simulink model "Microgrid_System"  (R2023b)
settings: Solver=ode23t  StartTime=0.0  StopTime=15.0  RelTol=1e-3
libraries: spsGroundLib x5, spsControlledCurrentSourceLib x4, eeGeneralControl x3, spsPowerLib x3, spsACVoltageSourceLib x1, spsCurrentMeasurementLib x1, spsParallelRLCLoadLib x1, spsSeriesRLCBranchLib x1, spsVoltageMeasurementLib x1, spspowerguiLib x1
settings Model: Creator=Ekta kumari khanda  LastModifiedBy=Ekta kumari khanda

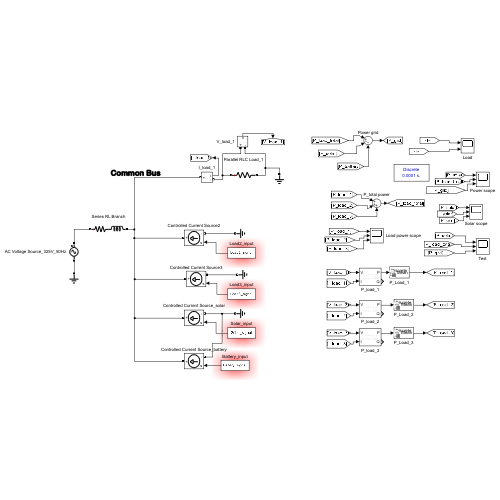
[thumbnail: Simulink's stored preview of the top-level diagram]
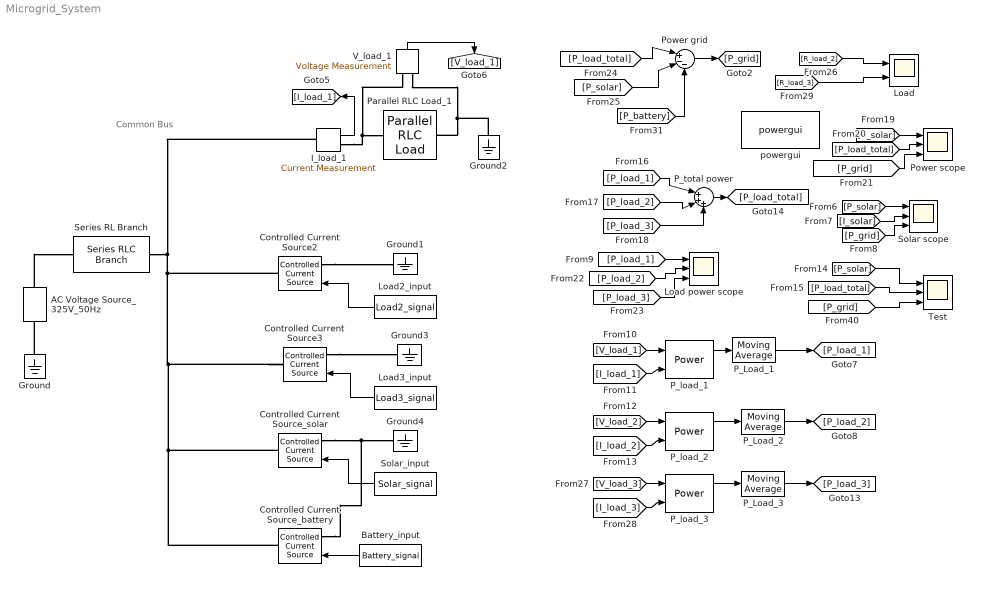
== system Microgrid_System ==
  note: Common Bus
  AC Voltage Source_325V_50Hz : spsACVoltageSourceLib/AC Voltage Source  Amplitude=325  Phase=0  Frequency=50  SampleTime=0  Measurements=None  BusType=swing  Pref=10e3  Qref=0  Qmin=-inf  Qmax=+inf
  Battery_input : FromWorkspace  VariableName=Battery_signal  SampleTime=-1  OutputAfterFinalValue=Holding final value
  Controlled Current Source2 : spsControlledCurrentSourceLib/Controlled Current Source  Initialize=on  Source_Type=AC  Amplitude=0  Phase=0  Frequency=0  Measurements=None
  Controlled Current Source3 : spsControlledCurrentSourceLib/Controlled Current Source  Initialize=on  Source_Type=AC  Amplitude=0  Phase=0  Frequency=0  Measurements=None
  Controlled Current Source_battery : spsControlledCurrentSourceLib/Controlled Current Source  Initialize=on  Source_Type=AC  Amplitude=0  Phase=0  Frequency=0  Measurements=None
  Controlled Current Source_solar : spsControlledCurrentSourceLib/Controlled Current Source  Initialize=on  Source_Type=AC  Amplitude=0  Phase=0  Frequency=0  Measurements=None
  Ground{,1..4} (5 alike) : spsGroundLib/Ground  LConnTagsString=a
  I_load_1 : spsCurrentMeasurementLib/Current Measurement  PhasorSimulation=off  OutputType=Complex  PSBequivalent=0
  Load : Scope  NumInputPorts=2
  Load power scope : Scope  NumInputPorts=3
  Load2_input : FromWorkspace  VariableName=Load2_signal  SampleTime=-1  OutputAfterFinalValue=Holding final value
  Load3_input : FromWorkspace  VariableName=Load3_signal  SampleTime=-1  OutputAfterFinalValue=Holding final value
  P_Load_1 : eeGeneralControl/Moving Average  VariantControl=Variant1  LabelModeActiveChoice=Discrete  f=50  x0=0  BufferSize=8192  Ts=0.001
      settings: LibrarySourceBlock=ee_sl_lib/General Control/Moving Average
  P_Load_2 : eeGeneralControl/Moving Average  VariantControl=Variant1  LabelModeActiveChoice=Discrete  f=50  x0=0  BufferSize=8192  Ts=0.001
      settings: LibrarySourceBlock=ee_sl_lib/General Control/Moving Average
  P_Load_3 : eeGeneralControl/Moving Average  VariantControl=Variant1  LabelModeActiveChoice=Discrete  f=50  x0=0  BufferSize=8192  Ts=0.001
      settings: LibrarySourceBlock=ee_sl_lib/General Control/Moving Average
  P_load_1 : spsPowerLib/Power  Freq=60  Vinit=[1, 0]  Iinit=[1, 0]  Ts=0
  P_load_2 : spsPowerLib/Power  Freq=60  Vinit=[1, 0]  Iinit=[1, 0]  Ts=0
  P_load_3 : spsPowerLib/Power  Freq=60  Vinit=[1, 0]  Iinit=[1, 0]  Ts=0
  P_total power : Sum  Inputs=|+++
  Parallel RLC Load_1 : spsParallelRLCLoadLib/Parallel RLC Load  LConnTagsString=a  RConnTagsString=__new0  NominalVoltage=230  NominalFrequency=50  ActivePower=1500  InductivePower=0  CapacitivePower=0  Setx0=off  InitialVoltage=0  SetiL0=off  InitialCurrent=0  Measurements=None  LoadType=constant Z
      settings: AttributesFormatString=\n  LibrarySourceBlock=sps_lib/Passives/Parallel RLC Load
  Power grid : Sum  Inputs=|+--
  Power scope : Scope  NumInputPorts=3
  Series RL Branch : spsSeriesRLCBranchLib/Series RLC Branch  LConnTagsString=__new0  RConnTagsString=__new0  BranchType=RL  Resistance=0.5  Inductance=1e-3  SetiL0=off  InitialCurrent=0  Capacitance=1e-6  Setx0=off  InitialVoltage=0  Measurements=None
  Solar scope : Scope  NumInputPorts=3
  Solar_input : FromWorkspace  VariableName=Solar_signal  SampleTime=-1  OutputAfterFinalValue=Holding final value
  Test : Scope  NumInputPorts=3
  V_load_1 : spsVoltageMeasurementLib/Voltage Measurement  PhasorSimulation=off  OutputType=Complex  PSBequivalent=0
  powergui : spspowerguiLib/powergui  Priority=1  SimulationMode=Discrete  SampleTime=0.0001  frequency=60  Iterations=50  frequencyindice=0  Pbase=100e6  ErrMax=1e-4  UnitsV=kV  UnitsW=MW  buscounter=0  FunctionMessages=off  echomessages=off  EnableUseOfTLC=off  CurrentSourceSwitches=off  DisableSnubberDevices=off  DisableRonSwitches=off  DisableVfSwitches=off  DisplayEquations=off  AutomaticDiscreteSolvers=off  SolverType=Tustin/Backward Euler (TBE)  Interpol=off  ExternalGateDelay=off  methode=off  Ts=100  x0status=blocks  SPID=on  SwTol=0  HookPort=off  NonlinearTolerance=1e-4  nMaxIteration=100  ContinueOnMaxIteration=off  RestoreLinks=warning  ResistiveCurrentMeasurement=off  Frange=[0:2:500]  Ylog=off  Xlog=on  ShowGrid=off  save=off  variable=ZData  structure=0  ZoomFFT=off  StartTime=0.0  cycles=1  DisplayStyle=1  fundamental=60  FreqAxis=off  MaxFrequency=1000  frequencyindicesteady=1  RmsSteady=1  display=off
  wires:
  [P_solar] -> Solar scope/1
  [P_grid] -> Solar scope/3
  [I_solar] -> Solar scope/2
  I_load_1/1 -> [I_load_1]
  V_load_1/1 -> [V_load_1]
  [I_load_1] -> P_load_1/2
  [V_load_1] -> P_load_1/1
  [V_load_2] -> P_load_2/1
  P_load_2/1 -> P_Load_2/1
  [I_load_2] -> P_load_2/2
  P_Load_2/1 -> [P_load_2]
  [P_load_1] -> P_total power/1
  [P_load_2] -> P_total power/2
  [P_load_3] -> P_total power/3
  P_total power/1 -> [P_load_total]
  [P_solar] -> Power scope/1
  [P_grid] -> Power scope/3
  [P_load_total] -> Power scope/2
  [P_load_3] -> Load power scope/3
  [P_load_2] -> Load power scope/2
  [P_load_1] -> Load power scope/1
  P_Load_1/1 -> [P_load_1]
  P_load_1/1 -> P_Load_1/1
  [P_load_total] -> Test/2
  [P_solar] -> Test/1
  [P_grid] -> Test/3
  P_Load_3/1 -> [P_load_3]
  [I_load_3] -> P_load_3/2
  P_load_3/1 -> P_Load_3/1
  [V_load_3] -> P_load_3/1
  [R_load_2] -> Load/1
  [R_load_3] -> Load/2
  Load2_input/1 -> Controlled Current Source2/1
  Load3_input/1 -> Controlled Current Source3/1
  Solar_input/1 -> Controlled Current Source_solar/1
  Power grid/1 -> [P_grid]
  [P_load_total] -> Power grid/1
  [P_solar] -> Power grid/2
  Battery_input/1 -> Controlled Current Source_battery/1
  [P_battery] -> Power grid/3
  connections:
  Ground/LConn1 -- AC Voltage Source_325V_50Hz/LConn1
  I_load_1/RConn1 -- Parallel RLC Load_1/LConn1 -- V_load_1/LConn1
  V_load_1/LConn2 -- Ground2/LConn1 -- Parallel RLC Load_1/RConn1
  AC Voltage Source_325V_50Hz/RConn1 -- Series RL Branch/LConn1
  Series RL Branch/RConn1 -- I_load_1/LConn1 -- Controlled Current Source_solar/RConn1 -- Controlled Current Source_battery/RConn1 -- Controlled Current Source3/RConn1 -- Controlled Current Source2/RConn1
  Controlled Current Source3/LConn1 -- Ground3/LConn1
  Controlled Current Source2/LConn1 -- Ground1/LConn1
  Controlled Current Source_solar/LConn1 -- Controlled Current Source_battery/LConn1 -- Ground4/LConn1
